simulink model "Active_Suspension_Sim"  (R2021a)
settings: Solver=FixedStepAuto  StartTime=0.0  StopTime=10  FixedStep=0.01  MaxStep=0.1  RelTol=1e-3
undefined symbols (not defined in the file): Actuator_Force, amplitude, Choice, Choice_Road_Profile, D, delay_time, final_value, Frequency, initial_output, initial_value, N, Slope, step_time
libraries: simulink x1
settings Model: Creator=ski_w  LastModifiedBy=DESKTOP-B6L2DB0
settings SolverCC: AlgebraicLoopSolver=TrustRegion
settings DataIOCC: SaveFormat=StructureWithTime
settings DebuggingCC: SFMachineParentedDataDiag=warning

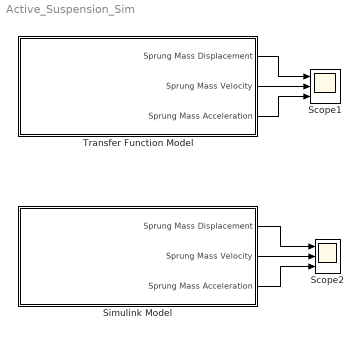
== system Active_Suspension_Sim ==
  Scope1 : Scope  NumInputPorts=3
  Scope2 : Scope  NumInputPorts=3
  Simulink Model : Subsystem
  Transfer Function Model : Subsystem
  wires:
  Simulink Model/1(Sprung Mass Displacement) -> Scope2/1
  Simulink Model/2(Sprung Mass Velocity) -> Scope2/2
  Simulink Model/3(Sprung Mass Acceleration) -> Scope2/3
  Transfer Function Model/1(Sprung Mass Displacement) -> Scope1/1
  Transfer Function Model/2(Sprung Mass Velocity) -> Scope1/2
  Transfer Function Model/3(Sprung Mass Acceleration) -> Scope1/3

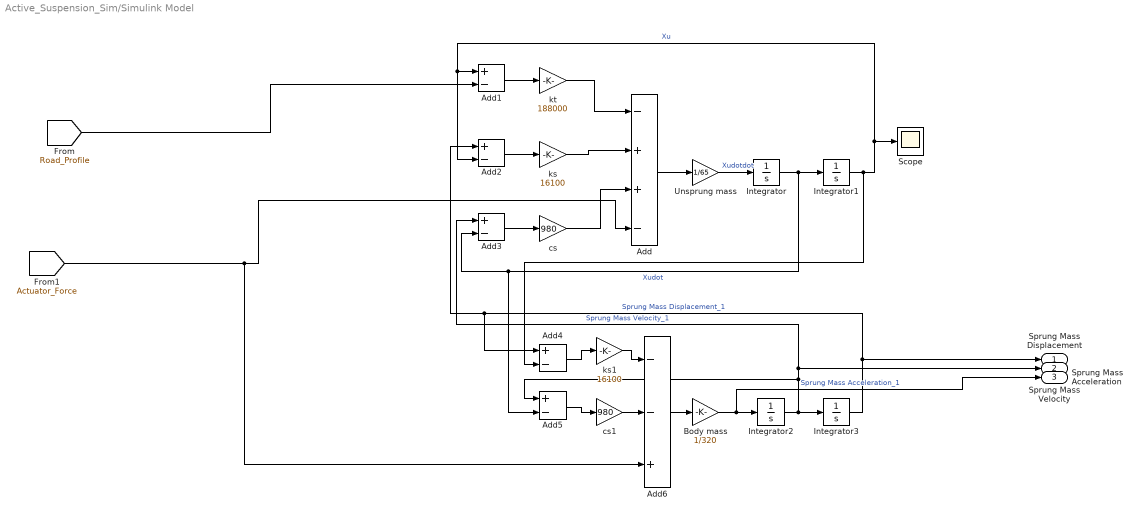
== system Active_Suspension_Sim/Simulink Model ==
  Add : Sum  Inputs=-++-
  Add{1..5} (5 alike) : Sum  Inputs=+-
  Add6 : Sum  Inputs=--+
  Body mass : Gain  Gain=1/320
  Integrator{,1..3} (4 alike) : Integrator
  Scope : Scope
  Unsprung mass : Gain  Gain=1/65
  cs : Gain  Gain=980
  cs1 : Gain  Gain=980
  ks : Gain  Gain=16100
  ks1 : Gain  Gain=16100
  kt : Gain  Gain=188000
  Sprung Mass Displacement : Outport
  Sprung Mass Velocity : Outport  Port=2
  Sprung Mass Acceleration : Outport  Port=3
  wires:
  Add/1 -> Unsprung mass/1
  Add3/1 -> cs/1
  Integrator/1 -> Integrator1/1, Add5/2, Add3/2  "Xudot"
  Integrator1/1 -> Scope/1, Add2/2, Add1/1, Add4/2  "Xu"
  Integrator3/1 -> Sprung Mass Displacement/1, Add4/1, Add2/1  "Sprung Mass Displacement_1"
  Add6/1 -> Body mass/1
  cs1/1 -> Add6/2
  Integrator2/1 -> Integrator3/1, Add5/1, Sprung Mass Velocity/1, Add3/1  "Sprung Mass Velocity_1"
  Add4/1 -> ks1/1
  ks/1 -> Add/2
  Add2/1 -> ks/1
  Add5/1 -> cs1/1
  ks1/1 -> Add6/1
  kt/1 -> Add/1
  Body mass/1 -> Sprung Mass Acceleration/1, Integrator2/1  "Sprung Mass Acceleration_1"
  cs/1 -> Add/3
  Unsprung mass/1 -> Integrator/1  "Xudotdot"
  Add1/1 -> kt/1
  [Road_Profile] -> Add1/2
  [Actuator_Force] -> Add6/3, Add/4

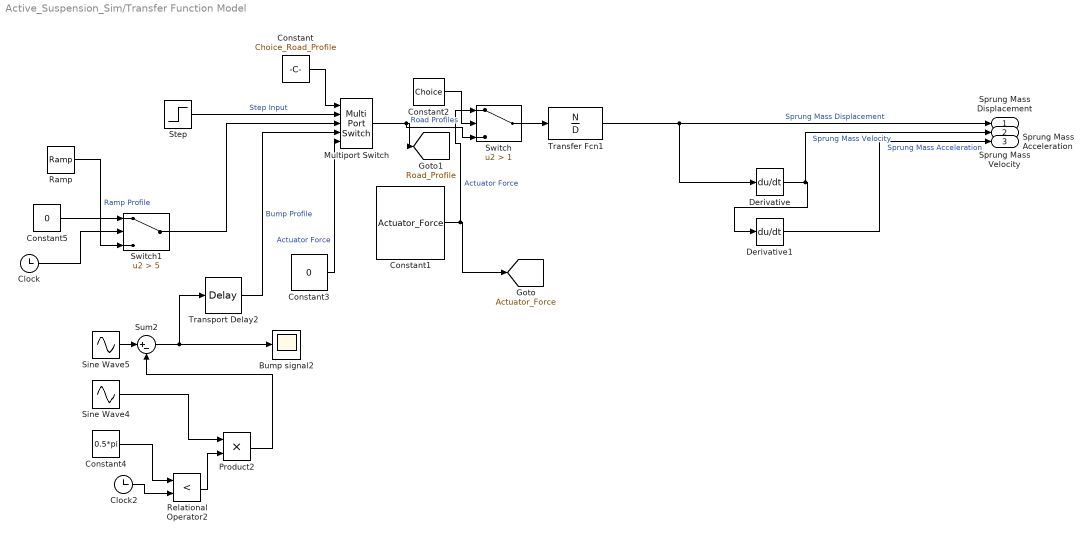
== system Active_Suspension_Sim/Transfer Function Model ==
  Bump signal2 : Scope
  Clock : Clock
  Clock2 : Clock
      settings: Decimation=100
  Constant : Constant  Value=Choice_Road_Profile  VectorParams1D=off
  Constant1 : Constant  Value=Actuator_Force
  Constant2 : Constant  Value=Choice
  Constant3 : Constant  Value=0
  Constant4 : Constant  Value=0.5*pi
  Constant5 : Constant  Value=0
  Derivative : Derivative
  Derivative1 : Derivative
  Multiport Switch : MultiPortSwitch  Inputs=4
  Product2 : Product
  Ramp : simulink/Sources/Ramp  slope=Slope  start=Start_time  InitialOutput=initial_output
  Relational Operator2 : RelationalOperator  Operator=<  OutDataTypeStr=boolean  RndMeth=Simplest
  Sine Wave4 : Sin  Amplitude=amplitude  Frequency=Frequency  SampleTime=0
  Sine Wave5 : Sin  Amplitude=amplitude  Frequency=Frequency  SampleTime=0
  Step : Step  Time=step_time  Before=initial_value  After=final_value  SampleTime=0
  Sum2 : Sum  Inputs=|+-
  Switch : Switch  Criteria=u2 > Threshold  Threshold=1
  Switch1 : Switch  Criteria=u2 > Threshold  Threshold=5
  Transfer Fcn1 : TransferFcn  Numerator=N  Denominator=D
  Transport Delay2 : TransportDelay  DelayTime=delay_time
  Sprung Mass Displacement : Outport
  Sprung Mass Velocity : Outport  Port=2
  Sprung Mass Acceleration : Outport  Port=3
  tag scope: Actuator_Force=global, Road_Profile=global
  wires:
  Switch/1 -> Transfer Fcn1/1
  Ramp/1 -> Switch1/3  "Ramp Profile"
  Transport Delay2/1 -> Multiport Switch/4  "Bump Profile"
  Constant2/1 -> Switch/2
  Multiport Switch/1 -> Switch/3, [Road_Profile]  "Road Profiles"
  Constant3/1 -> Multiport Switch/5  "Actuator Force"
  Derivative/1 -> Sprung Mass Velocity/1, Derivative1/1  "Sprung Mass Velocity"
  Step/1 -> Multiport Switch/2  "Step Input"
  Constant1/1 -> Switch/1, [Actuator_Force]  "Actuator Force"
  Constant4/1 -> Relational Operator2/1
  Sine Wave5/1 -> Sum2/1
  Derivative1/1 -> Sprung Mass Acceleration/1  "Sprung Mass Acceleration"
  Clock2/1 -> Relational Operator2/2
  Transfer Fcn1/1 -> Sprung Mass Displacement/1, Derivative/1  "Sprung Mass Displacement"
  Product2/1 -> Sum2/2
  Constant/1 -> Multiport Switch/1
  Sum2/1 -> Transport Delay2/1, Bump signal2/1
  Sine Wave4/1 -> Product2/1
  Relational Operator2/1 -> Product2/2
  Constant5/1 -> Switch1/1
  Switch1/1 -> Multiport Switch/3
  Clock/1 -> Switch1/2
